simulink model "SMC_Vs_DSMC"  (R2019b)
settings: Solver=VariableStepAuto  StartTime=0.0  StopTime=100  RelTol=1e-3
settings Model: Creator=Asus  LastModifiedBy=Asus

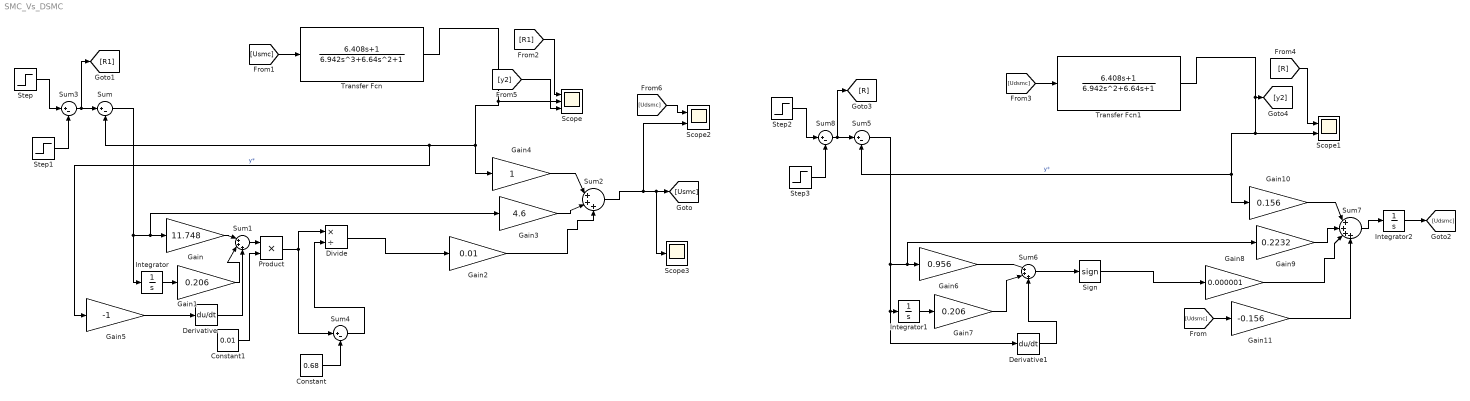
== system SMC_Vs_DSMC ==
  Constant : Constant  Value=0.68
  Constant1 : Constant  Value=0.01
  Derivative : Derivative
  Derivative1 : Derivative
  Divide : Product  Inputs=*/
  Gain : Gain  Gain=11.748
  Gain1 : Gain  Gain=0.206
  Gain10 : Gain  Gain=0.156
  Gain11 : Gain  Gain=-0.156
  Gain2 : Gain  Gain=0.01
  Gain3 : Gain  Gain=4.6
  Gain4 : Gain
  Gain5 : Gain  Gain=-1
  Gain6 : Gain  Gain=0.956
  Gain7 : Gain  Gain=0.206
  Gain8 : Gain  Gain=0.000001
  Gain9 : Gain  Gain=0.2232
  Integrator : Integrator
  Integrator1 : Integrator
  Integrator2 : Integrator
  Product : Product
  Scope : Scope  NumInputPorts=3
  Scope1 : Scope  NumInputPorts=2
  Scope2 : Scope  NumInputPorts=2
  Scope3 : Scope
  Sign : Signum
  Step : Step  Time=5  SampleTime=0
  Step1 : Step  Time=60  After=0.5  SampleTime=0
  Step2 : Step  Time=5  SampleTime=0
  Step3 : Step  Time=60  After=0.5  SampleTime=0
  Sum{,3..5,8} (5 alike) : Sum  Inputs=|+-
  Sum1 : Sum  Inputs=|+++
  Sum2 : Sum  Inputs=|+++
  Sum6 : Sum  Inputs=|+++
  Sum7 : Sum  Inputs=|++++
  Transfer Fcn : TransferFcn  Numerator=[6.408 1]  Denominator=[6.942 6.64 0 1]
  Transfer Fcn1 : TransferFcn  Numerator=[6.408 1]  Denominator=[6.942 6.64 1]
  wires:
  Sum1/1 -> Product/1
  Gain3/1 -> Sum2/2
  Transfer Fcn/1 -> Gain5/1, Sum/2, Gain4/1, Scope/2  "y*"
  Gain4/1 -> Sum2/1
  Gain2/1 -> Sum2/3
  Step1/1 -> Sum3/2
  [Usmc] -> Transfer Fcn/1
  [R1] -> Scope/1
  Gain/1 -> Sum1/1
  Sum4/1 -> Divide/2
  Gain5/1 -> Derivative/1
  Product/1 -> Divide/1, Sum4/1
  Constant/1 -> Sum4/2
  Divide/1 -> Gain2/1
  Integrator/1 -> Gain1/1
  Derivative/1 -> Sum1/3
  Gain1/1 -> Sum1/2
  Sum/1 -> Gain3/1, Gain/1, Integrator/1
  Sum3/1 -> [R1], Sum/1
  Constant1/1 -> Product/2
  Step/1 -> Sum3/1
  Sum2/1 -> Scope2/2, Scope3/1, [Usmc]
  Step2/1 -> Sum8/1
  Sum8/1 -> [R], Sum5/1
  Sum5/1 -> Gain9/1, Gain6/1, Derivative1/1, Integrator1/1
  Sign/1 -> Gain8/1
  Gain7/1 -> Sum6/2
  Derivative1/1 -> Sum6/3
  Integrator1/1 -> Gain7/1
  Gain11/1 -> Sum7/4
  Gain6/1 -> Sum6/1
  Sum6/1 -> Sign/1
  [R] -> Scope1/1
  Integrator2/1 -> [Udsmc]
  [Udsmc] -> Gain11/1
  Step3/1 -> Sum8/2
  [Udsmc] -> Transfer Fcn1/1
  Sum7/1 -> Integrator2/1
  Gain10/1 -> Sum7/1
  Gain8/1 -> Sum7/3
  Gain9/1 -> Sum7/2
  Transfer Fcn1/1 -> Scope1/2, Sum5/2, Gain10/1, [y2]  "y*"
  [y2] -> Scope/3
  [Udsmc] -> Scope2/1
